simulink model "CircuitoRC_simulink"  (R2022b)
settings: Solver=VariableStepAuto  StartTime=0.0  StopTime=10.0  RelTol=1e-3
values from neighbouring files (symbols this model uses):
  C = 1*10^-3    (= 0.001)    [CircuitoRC.m]    (also in CircuitoRC_SS.m = [1])
  R = 470    [CircuitoRC.m]    (also in CircuitoRC_SS.m)
settings Model: Creator=giuli  LastModifiedBy=giuli

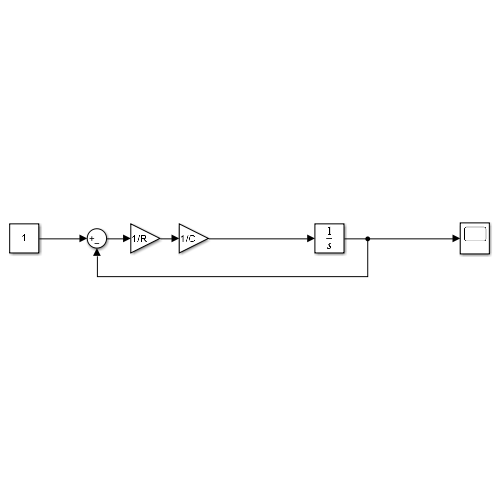
[thumbnail: Simulink's stored preview of the top-level diagram]
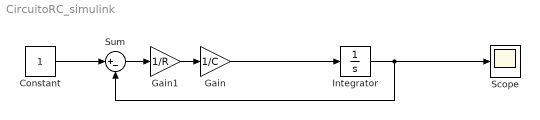
== system CircuitoRC_simulink ==
  Constant : Constant
  Gain : Gain  Gain=1/C
  Gain1 : Gain  Gain=1/R
  Integrator : Integrator
  Scope : Scope
  Sum : Sum  Inputs=|+-
  wires:
  Gain/1 -> Integrator/1
  Gain1/1 -> Gain/1
  Sum/1 -> Gain1/1
  Integrator/1 -> Scope/1, Sum/2
  Constant/1 -> Sum/1
